simulink model "servoUpperSim"  (R2022b)
settings: Solver=VariableStepAuto  StartTime=0.0  StopTime=5  RelTol=1e-8
settings Model: Creator=HP  LastModifiedBy=HP
settings SolverCC: AlgebraicLoopSolver=TrustRegion
settings DebuggingCC: UnconnectedInputMsg=warning  UnconnectedOutputMsg=warning  UnconnectedLineMsg=warning  SFMachineParentedDataDiag=warning
settings ModelReferenceCC: EnableRefExpFcnMdlSchedulingChecks=on
settings RTWCC: DLArmComputeVersion=19.05

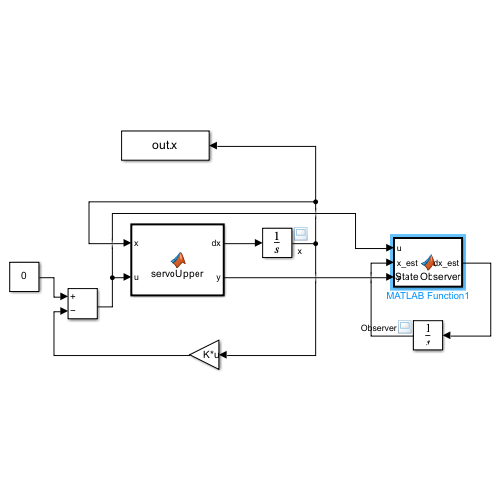
[thumbnail: Simulink's stored preview of the top-level diagram]
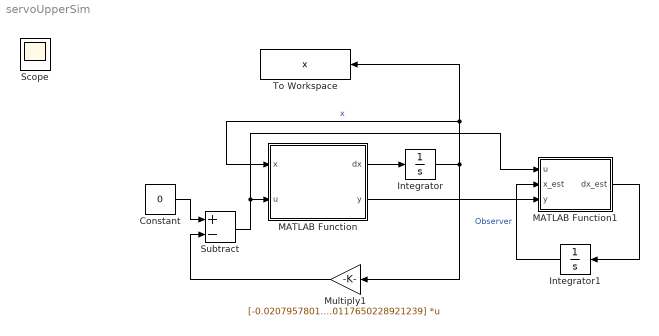
== system servoUpperSim ==
  Constant : Constant  Value=0
  Integrator : Integrator  InitialCondition=[0; 0.1; 0; 0]  IgnoreLimit=on
  Integrator1 : Integrator  InitialCondition=[0; 0.1; 0; 0]
  MATLAB Function : MATLAB Function  TreatAsAtomicUnit=on
  MATLAB Function1 : MATLAB Function  TreatAsAtomicUnit=on
  Multiply1 : Gain  Gain="[-0.0207957801019633\t0.143430567548806\t-0.00777706617299729\t0.0117650228921239]"  Multiplication=Matrix(K*u)
  Subtract : Sum  Inputs=+-
  To Workspace : ToWorkspace  VariableName=x  SaveFormat=Timeseries  SampleTime=-1
  Scope : Scope
  wires:
  Constant/1 -> Subtract/1
  MATLAB Function/1(dx) -> Integrator/1
  Integrator/1 -> Multiply1/1, To Workspace/1, MATLAB Function/1(x)  "x"
  Multiply1/1 -> Subtract/2
  Subtract/1 -> MATLAB Function1/1(u), MATLAB Function/2(u)
  MATLAB Function1/1(dx_est) -> Integrator1/1
  Integrator1/1 -> MATLAB Function1/2(x_est)  "Observer"
  MATLAB Function/2(y) -> MATLAB Function1/3(y)

== matlab function servoUpperSim/MATLAB Function1 ==
  data: u input; dx_est output; x_est input; y input
function dx_est  = StateObserver(u,x_est,y)
F = [-13.6162    0.5990    1.0000         0;
     3.8834  -25.3861         0    1.0000;
    -3.7884    7.8602  -10.1274   -0.5005;
    54.6516 -155.1368  -10.0097   -0.8702];


B=[ 0;
    0;
    10127.4369;
    10009.6760];

L= [13.6162   -0.5990;
   -3.8834   25.3861;
    3.7884  144.1456;
  -54.6516  419.4448];

dx_est=F*x_est+L*y+B*u;

== matlab function servoUpperSim/MATLAB Function ==
  data: x input; u input; dx output; y output
function [dx,y] = servoUpper(x,u)
%% Motor
% Resistance
Rm = 8.4;
% Current-torque (N-m/A)
kt = 0.042;
% Back-emf constant (V-s/rad)
km = 0.042;
%
%% Rotary Arm
% Mass (kg)
mr = 0.095;
% Total length (m)
r = 0.085;
% Moment of inertia about pivot (kg-m^2)
Jr = mr*r^2/3;
% Equivalent Viscous Damping Coefficient (N-m-s/rad)
br = 1e-3; % damping tuned heuristically to match QUBE-Sero 2 response
%
%% Pendulum Link
% Mass (kg)
mp = 0.024;
% Total length (m)
Lp = 0.129;
% Pendulum center of mass (m)
l = Lp/2;
% Moment of inertia about pivot (kg-m^2)
Jp = mp*Lp^2/3;
% Equivalent Viscous Damping Coefficient (N-m-s/rad)
bp = 5e-5; % damping tuned heuristically to match QUBE-Sero 2 response
% Gravity Constant
g = 9.81;
Jt=Jp*Jr-mp^2*l^2*r^2;
%Control voltage and the torque
%%
% state vectors 

%%
Jt = Jr*Jp - mp^2*r^2*l^2;
% State Space Representation
A = [0 0 1 0;
     0 0 0 1;
     0 mp^2*l^2*r*g/Jt  -br*Jp/Jt   -mp*l*r*bp/Jt 
     0  mp*g*l*Jr/Jt    -mp*l*r*br/Jt   -Jr*bp/Jt];

B=[0; 0; Jp/Jt; mp*r*l/Jt];
C=[1 0 0 0;
   0 1 0 0];
D=[0 ; 0];
dx=A*x+B.*u;
y=C*x+D.*u;
